simulink model "tcpsimtest"  (R2022a)
settings: Solver=VariableStepAuto  StartTime=0.0  StopTime=10.0  RelTol=1e-3
libraries: instrumentlib x2
settings Model: Creator=user  LastModifiedBy=user

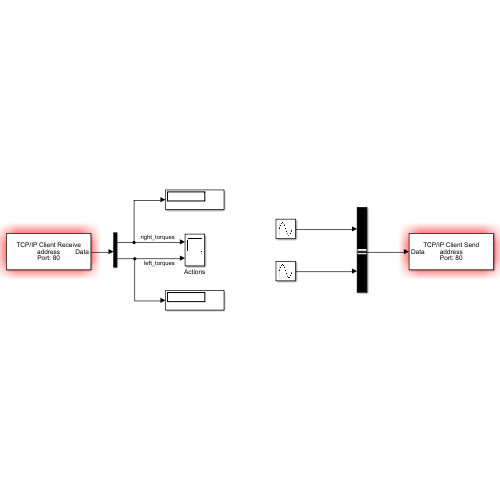
[thumbnail: Simulink's stored preview of the top-level diagram]
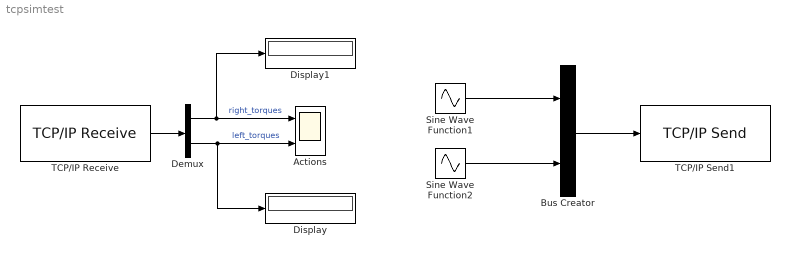
== system tcpsimtest ==
  Actions : Scope  NumInputPorts=2
  Bus Creator : BusCreator  Inputs=2
  Demux : Demux  Outputs=2
  Display : Display
  Display1 : Display
  Sine Wave Function1 : Sin  Amplitude=10  SampleTime=0
  Sine Wave Function2 : Sin  Amplitude=10  Phase=90  SampleTime=0
  TCP/IP Receive : instrumentlib/TCP//IP Receive  Host=address  Port=port  DataSize=[ 1, 1 ]  DataType=uint8  ASCIIFormatting=%f  Terminator=LF  CustomTerminator=10  ByteOrder=big-endian  EnableBlockingMode=on  Timeout=10  SampleTime=0.01  SimulateUsing=Interpreted execution
  TCP/IP Send1 : instrumentlib/TCP//IP Send  Host=address  Port=port  ByteOrder=big-endian  EnableBlockingMode=on  Timeout=100  TransferDelay=on  SimulateUsing=Interpreted execution
  wires:
  Demux/1 -> Actions/1, Display1/1  "right_torques"
  TCP/IP Receive/1 -> Demux/1
  Demux/2 -> Display/1, Actions/2  "left_torques"
  Bus Creator/1 -> TCP/IP Send1/1
  Sine Wave Function2/1 -> Bus Creator/2
  Sine Wave Function1/1 -> Bus Creator/1
